simulink model "boostConverter"  (R2021a)
settings: Solver=VariableStepAuto  StartTime=0.0  StopTime=1  RelTol=1e-3
undefined symbols (not defined in the file): C, L
libraries: spsSeriesRLCBranchLib x6, spsCurrentMeasurementLib x4, spsMosfetLib x3, spsDCVoltageSourceLib x2, spsVoltageMeasurementLib x2, spsDiodeLib x1, simulink x1, spspowerguiLib x1
settings Model: Creator=User  LastModifiedBy=User

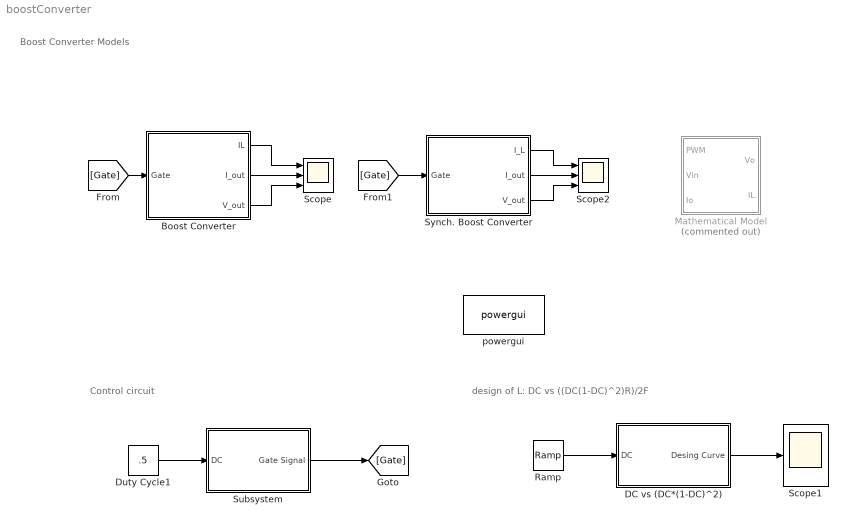
== system boostConverter ==
  note: Control circuit
  note: Boost Converter Models
  note: design of L: DC vs ((DC(1-DC)^2)R)/2F
  " DC vs (DC*(1-DC)^2) " : Subsystem  mask{F=50000, R=10, L=1e-5}
  Boost Converter : Subsystem
  Duty Cycle1 : Constant  Value=.5
  Mathematical Model : Subsystem  Commented=on
  Ramp : simulink/Sources/Ramp  slope=1  start=0  InitialOutput=0
  Scope : Scope  NumInputPorts=3
  Scope1 : Scope
  Scope2 : Scope  NumInputPorts=3
  Subsystem : Subsystem
  Synch. Boost Converter : Subsystem
  powergui : spspowerguiLib/powergui  Priority=1  SimulationMode=Continuous  SampleTime=50e-6  frequency=60  Iterations=50  frequencyindice=0  Pbase=100e6  ErrMax=1e-4  UnitsV=kV  UnitsW=MW  buscounter=0  FunctionMessages=off  echomessages=off  EnableUseOfTLC=off  CurrentSourceSwitches=off  DisableSnubberDevices=off  DisableRonSwitches=off  DisableVfSwitches=off  DisplayEquations=off  AutomaticDiscreteSolvers=off  SolverType=Tustin/Backward Euler (TBE)  Interpol=off  ExternalGateDelay=off  methode=off  Ts=100  x0status=blocks  SPID=on  SwTol=0  HookPort=off  NonlinearTolerance=1e-4  nMaxIteration=100  ContinueOnMaxIteration=off  RestoreLinks=warning  ResistiveCurrentMeasurement=off  Frange=[0:2:500]  Ylog=off  Xlog=on  ShowGrid=off  save=off  variable=ZData  structure=0  ZoomFFT=off  StartTime=0.0  cycles=1  DisplayStyle=1  fundamental=60  FreqAxis=off  MaxFrequency=1000  frequencyindicesteady=1  RmsSteady=1  display=off
  wires:
  Duty Cycle1/1 -> Subsystem/1(DC)
  [Gate] -> Boost Converter/1(Gate)
  Subsystem/1(Gate Signal) -> [Gate]
  Ramp/1 -> " DC vs (DC*(1-DC)^2) "/1(DC)
  " DC vs (DC*(1-DC)^2) "/1(Desing Curve) -> Scope1/1
  Boost Converter/1(IL) -> Scope/1
  Boost Converter/2(I_out) -> Scope/2
  Boost Converter/3(V_out) -> Scope/3
  [Gate] -> Synch. Boost Converter/1(Gate)
  Synch. Boost Converter/2(I_out) -> Scope2/2
  Synch. Boost Converter/1(I_L) -> Scope2/1
  Synch. Boost Converter/3(V_out) -> Scope2/3

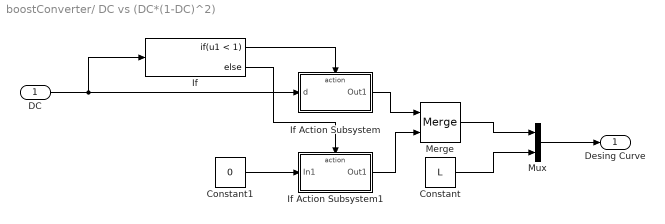
== system boostConverter/ DC vs (DC*(1-DC)^2)  ==
  DC : Inport
  Constant : Constant  Value=L
  Constant1 : Constant  Value=0
  If : If  IfExpression=u1 < 1
  If Action Subsystem : Subsystem  TreatAsAtomicUnit=on
  If Action Subsystem1 : Subsystem  TreatAsAtomicUnit=on
  Merge : Merge
  Mux : Mux  Inputs=2
  Desing Curve : Outport
  wires:
  Constant1/1 -> If Action Subsystem1/1(In1)
  If Action Subsystem/1(Out1) -> Merge/1
  If Action Subsystem1/1(Out1) -> Merge/2
  If/1 -> If Action Subsystem/Action
  DC/1 -> If/1, If Action Subsystem/1(d)
  If/2 -> If Action Subsystem1/Action
  Merge/1 -> Mux/1
  Constant/1 -> Mux/2
  Mux/1 -> Desing Curve/1

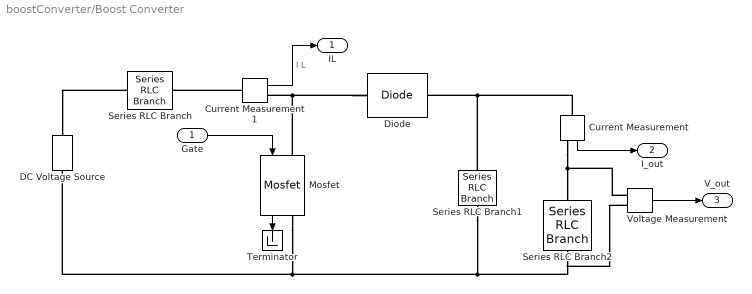
== system boostConverter/Boost Converter ==
  Gate : Inport
  Current Measurement : spsCurrentMeasurementLib/Current Measurement  PhasorSimulation=off  OutputType=Complex  PSBequivalent=0
  Current Measurement1 : spsCurrentMeasurementLib/Current Measurement  PhasorSimulation=off  OutputType=Complex  PSBequivalent=0
  DC Voltage Source : spsDCVoltageSourceLib/DC Voltage Source  Amplitude=100  Measurements=None
  Diode : spsDiodeLib/Diode  Ron=0.001  Lon=0  Vf=0.8  IC=0  UseSnubber=0  Rs=500  Cs=250e-9  Measurements=off
  Mosfet : spsMosfetLib/Mosfet  Ron=0.1  Lon=0  Rd=0.01  Vfd=0  IC=0  Rs=1e5  Cs=inf  Measurements=on
  Series RLC Branch : spsSeriesRLCBranchLib/Series RLC Branch  LConnTagsString=__new0  RConnTagsString=__new0  BranchType=L  Resistance=1  Inductance=1e-5  SetiL0=off  InitialCurrent=0  Capacitance=1e-6  Setx0=off  InitialVoltage=0  Measurements=None
  Series RLC Branch1 : spsSeriesRLCBranchLib/Series RLC Branch  LConnTagsString=__new0  RConnTagsString=__new0  BranchType=C  Resistance=1  Inductance=1e-3  SetiL0=off  InitialCurrent=0  Capacitance=10e-3  Setx0=off  InitialVoltage=0  Measurements=None
  Series RLC Branch2 : spsSeriesRLCBranchLib/Series RLC Branch  LConnTagsString=__new0  RConnTagsString=__new0  BranchType=R  Resistance=10  Inductance=1e-3  SetiL0=off  InitialCurrent=0  Capacitance=1e-6  Setx0=off  InitialVoltage=0  Measurements=None
  Terminator : Terminator
  Voltage Measurement : spsVoltageMeasurementLib/Voltage Measurement  PhasorSimulation=off  OutputType=Complex  PSBequivalent=0
  IL : Outport
  I_out : Outport  Port=2
  V_out : Outport  Port=3
  wires:
  Gate/1 -> Mosfet/1
  Current Measurement/1 -> I_out/1
  Mosfet/1 -> Terminator/1
  Current Measurement1/1 -> IL/1  "I L"
  Voltage Measurement/1 -> V_out/1
  connections:
  Voltage Measurement/LConn2 -- Series RLC Branch2/RConn1 -- Series RLC Branch1/RConn1 -- Mosfet/RConn1 -- DC Voltage Source/LConn1
  Diode/LConn1 -- Mosfet/LConn1 -- Current Measurement1/RConn1
  Series RLC Branch1/LConn1 -- Current Measurement/LConn1 -- Diode/RConn1
  Current Measurement/RConn1 -- Series RLC Branch2/LConn1 -- Voltage Measurement/LConn1
  Current Measurement1/LConn1 -- Series RLC Branch/RConn1
  Series RLC Branch/LConn1 -- DC Voltage Source/RConn1

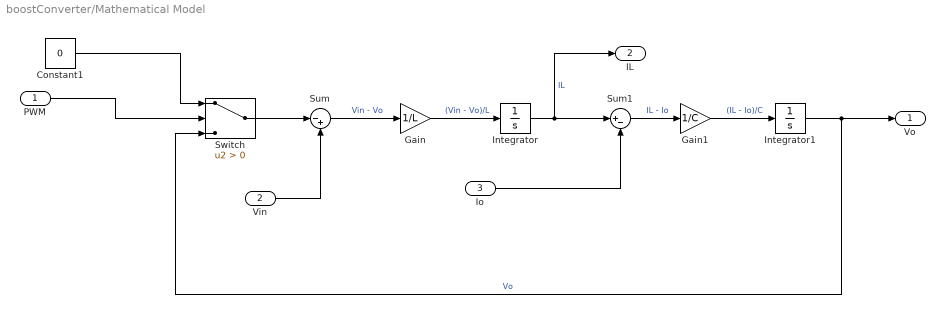
== system boostConverter/Mathematical Model ==
  PWM : Inport
  Vin : Inport  Port=2
  Io : Inport  Port=3
  Constant1 : Constant  Value=0
  Gain : Gain  Gain=1/L
  Gain1 : Gain  Gain=1/C
  Integrator : Integrator
  Integrator1 : Integrator
  Sum : Sum  Inputs=|-+
  Sum1 : Sum  Inputs=|+-
  Switch : Switch  Criteria=u2 > Threshold
  Vo : Outport
  IL : Outport  Port=2
  wires:
  Integrator1/1 -> Vo/1, Switch/3  "Vo"
  Vin/1 -> Sum/2
  Gain/1 -> Integrator/1  "(Vin - Vo)/L"
  Io/1 -> Sum1/2
  Constant1/1 -> Switch/1
  Gain1/1 -> Integrator1/1  "(IL - Io)/C"
  Integrator/1 -> IL/1, Sum1/1  "IL"
  Sum1/1 -> Gain1/1  "IL - Io"
  Sum/1 -> Gain/1  "Vin - Vo"
  Switch/1 -> Sum/1
  PWM/1 -> Switch/2

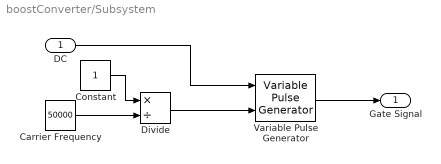
== system boostConverter/Subsystem ==
  DC : Inport
  Carrier Frequency : Constant  Value=50000
  Constant : Constant
  Divide : Product  Inputs=*/
  Variable Pulse Generator : VariablePulseGenerator  SampleTime=0.1
  Gate Signal : Outport
  wires:
  Constant/1 -> Divide/1
  Divide/1 -> Variable Pulse Generator/2
  DC/1 -> Variable Pulse Generator/1
  Variable Pulse Generator/1 -> Gate Signal/1
  Carrier Frequency/1 -> Divide/2

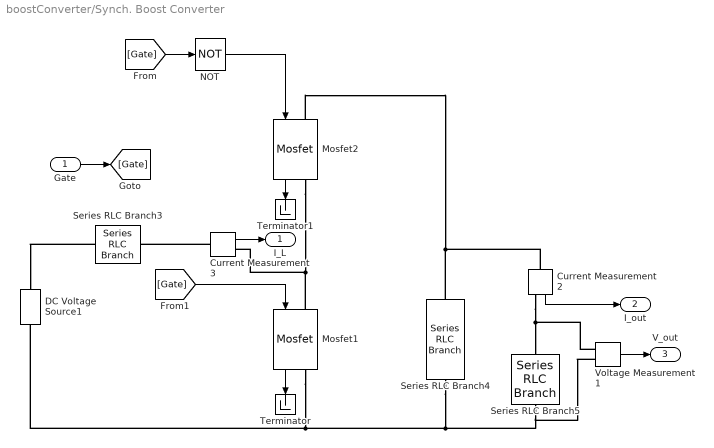
== system boostConverter/Synch. Boost Converter ==
  Gate : Inport
  Current Measurement2 : spsCurrentMeasurementLib/Current Measurement  PhasorSimulation=off  OutputType=Complex  PSBequivalent=0
  Current Measurement3 : spsCurrentMeasurementLib/Current Measurement  PhasorSimulation=off  OutputType=Complex  PSBequivalent=0
  DC Voltage Source1 : spsDCVoltageSourceLib/DC Voltage Source  Amplitude=100  Measurements=None
  Mosfet1 : spsMosfetLib/Mosfet  Ron=0.1  Lon=0  Rd=0.01  Vfd=0  IC=0  Rs=1e5  Cs=inf  Measurements=on
  Mosfet2 : spsMosfetLib/Mosfet  Ron=0.1  Lon=0  Rd=0.01  Vfd=0  IC=0  Rs=1e5  Cs=inf  Measurements=on
  NOT : Logic  Operator=NOT  IconShape=distinctive  AllPortsSameDT=off  OutDataTypeStr=boolean
  Series RLC Branch3 : spsSeriesRLCBranchLib/Series RLC Branch  LConnTagsString=__new0  RConnTagsString=__new0  BranchType=L  Resistance=1  Inductance=100e-3  SetiL0=off  InitialCurrent=0  Capacitance=1e-6  Setx0=off  InitialVoltage=0  Measurements=None
  Series RLC Branch4 : spsSeriesRLCBranchLib/Series RLC Branch  LConnTagsString=__new0  RConnTagsString=__new0  BranchType=C  Resistance=1  Inductance=1e-3  SetiL0=off  InitialCurrent=0  Capacitance=10e-3  Setx0=off  InitialVoltage=0  Measurements=None
  Series RLC Branch5 : spsSeriesRLCBranchLib/Series RLC Branch  LConnTagsString=__new0  RConnTagsString=__new0  BranchType=R  Resistance=10  Inductance=1e-3  SetiL0=off  InitialCurrent=0  Capacitance=1e-6  Setx0=off  InitialVoltage=0  Measurements=None
  Terminator : Terminator
  Terminator1 : Terminator
  Voltage Measurement1 : spsVoltageMeasurementLib/Voltage Measurement  PhasorSimulation=off  OutputType=Complex  PSBequivalent=0
  I_L : Outport
  I_out : Outport  Port=2
  V_out : Outport  Port=3
  wires:
  Voltage Measurement1/1 -> V_out/1
  NOT/1 -> Mosfet2/1
  Current Measurement2/1 -> I_out/1
  Current Measurement3/1 -> I_L/1
  Mosfet1/1 -> Terminator/1
  Mosfet2/1 -> Terminator1/1
  Gate/1 -> [Gate]
  [Gate] -> NOT/1
  [Gate] -> Mosfet1/1
  connections:
  Mosfet1/RConn1 -- DC Voltage Source1/LConn1 -- Series RLC Branch4/RConn1 -- Series RLC Branch5/RConn1 -- Voltage Measurement1/LConn2
  Series RLC Branch3/LConn1 -- DC Voltage Source1/RConn1
  Mosfet1/LConn1 -- Mosfet2/RConn1 -- Current Measurement3/RConn1
  Series RLC Branch4/LConn1 -- Mosfet2/LConn1 -- Current Measurement2/LConn1
  Current Measurement2/RConn1 -- Voltage Measurement1/LConn1 -- Series RLC Branch5/LConn1
  Current Measurement3/LConn1 -- Series RLC Branch3/RConn1

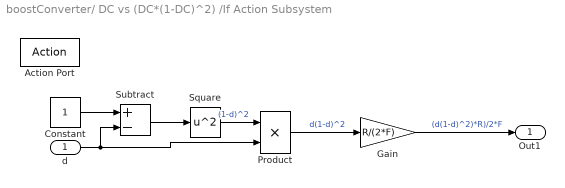
== system boostConverter/ DC vs (DC*(1-DC)^2) /If Action Subsystem ==
  d : Inport
  Action Port : ActionPort  ActionPortLabel=if(u1 < 1)
  Constant : Constant
  Gain : Gain  Gain=R/(2*F)
  Product : Product
  Square : Math  Operator=square  SaturateOnIntegerOverflow=on
  Subtract : Sum  Inputs=+-
  Out1 : Outport
  wires:
  d/1 -> Product/2, Subtract/2
  Subtract/1 -> Square/1
  Product/1 -> Gain/1  "d(1-d)^2"
  Square/1 -> Product/1  "(1-d)^2"
  Constant/1 -> Subtract/1
  Gain/1 -> Out1/1  "(d(1-d)^2)*R)/2*F"

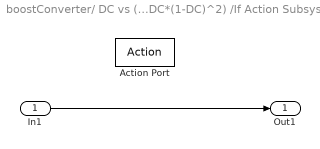
== system boostConverter/ DC vs (DC*(1-DC)^2) /If Action Subsystem1 ==
  In1 : Inport
  Action Port : ActionPort  ActionPortLabel=else
  Out1 : Outport
  wires:
  In1/1 -> Out1/1
